simulink model "SPWM"  (R2019b)
settings: Solver=VariableStepAuto  StartTime=0.0  StopTime=1  RelTol=1e-3
InitFcn:
  | Vd = 600
libraries: powerlib_meascontrol x4
settings Model: Creator=kanth  LastModifiedBy=kanth

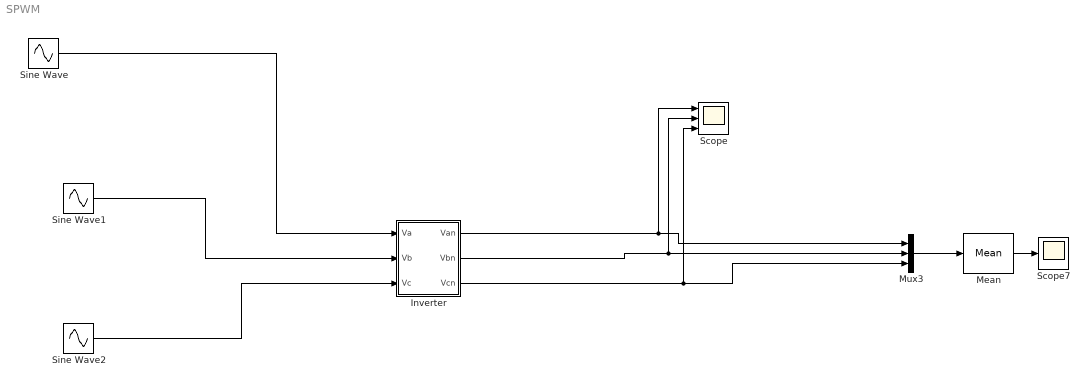
== system SPWM ==
  Inverter : Subsystem
  Mean : powerlib_meascontrol/Measurements/Mean  Freq=5000  Vinit=0  Ts=0
      settings: SourceProductName=Simscape Electrical
  Mux3 : Mux  Inputs=3
  Scope : Scope  NumInputPorts=3
  Scope7 : Scope
  Sine Wave : Sin  Amplitude=0.8  Frequency=314.159265  SampleTime=0
  Sine Wave1 : Sin  Amplitude=0.8  Frequency=314.159265  Phase=-2*pi/3  SampleTime=0
  Sine Wave2 : Sin  Amplitude=0.8  Frequency=314.159265  Phase=2*pi/3  SampleTime=0
  wires:
  Mux3/1 -> Mean/1
  Mean/1 -> Scope7/1
  Sine Wave/1 -> Inverter/1(Va)
  Sine Wave1/1 -> Inverter/2(Vb)
  Sine Wave2/1 -> Inverter/3(Vc)
  Inverter/1(Van) -> Scope/1, Mux3/1
  Inverter/2(Vbn) -> Scope/2, Mux3/2
  Inverter/3(Vcn) -> Scope/3, Mux3/3

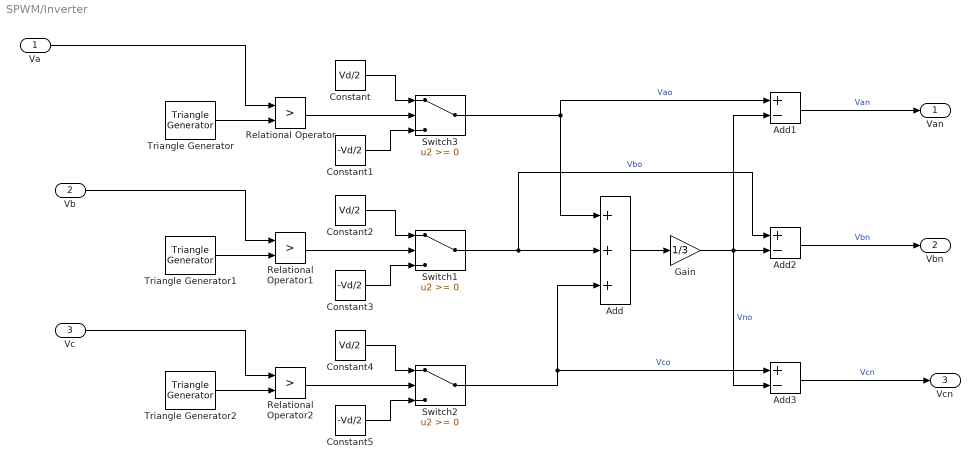
== system SPWM/Inverter ==
  Va : Inport
  Vb : Inport  Port=2
  Vc : Inport  Port=3
  Add : Sum  Inputs=+++
  Add1 : Sum  Inputs=+-
  Add2 : Sum  Inputs=+-
  Add3 : Sum  Inputs=+-
  Constant : Constant  Value=Vd/2
  Constant1 : Constant  Value=-Vd/2
  Constant2 : Constant  Value=Vd/2
  Constant3 : Constant  Value=-Vd/2
  Constant4 : Constant  Value=Vd/2
  Constant5 : Constant  Value=-Vd/2
  Gain : Gain  Gain=1/3
  Relational Operator : RelationalOperator  Operator=>  OutDataTypeStr=boolean  RndMeth=Simplest
  Relational Operator1 : RelationalOperator  Operator=>  OutDataTypeStr=boolean  RndMeth=Simplest
  Relational Operator2 : RelationalOperator  Operator=>  OutDataTypeStr=boolean  RndMeth=Simplest
  Switch1 : Switch
  Switch2 : Switch
  Switch3 : Switch
  Triangle Generator : powerlib_meascontrol/Pulse & Signal Generators/Triangle Generator  Freq=5000  Phase=0  Ts=0
      settings: SourceProductName=Simscape Electrical
  Triangle Generator1 : powerlib_meascontrol/Pulse & Signal Generators/Triangle Generator  Freq=5000  Phase=0  Ts=0
      settings: SourceProductName=Simscape Electrical
  Triangle Generator2 : powerlib_meascontrol/Pulse & Signal Generators/Triangle Generator  Freq=5000  Phase=0  Ts=0
      settings: SourceProductName=Simscape Electrical
  Van : Outport
  Vbn : Outport  Port=2
  Vcn : Outport  Port=3
  wires:
  Relational Operator1/1 -> Switch1/2
  Switch3/1 -> Add1/1, Add/1  "Vao"
  Switch1/1 -> Add/2, Add2/1  "Vbo"
  Constant2/1 -> Switch1/1
  Constant/1 -> Switch3/1
  Gain/1 -> Add3/2, Add2/2, Add1/2  "Vno"
  Constant3/1 -> Switch1/3
  Switch2/1 -> Add/3, Add3/1  "Vco"
  Relational Operator/1 -> Switch3/2
  Add3/1 -> Vcn/1  "Vcn"
  Triangle Generator/1 -> Relational Operator/2
  Triangle Generator2/1 -> Relational Operator2/2
  Constant1/1 -> Switch3/3
  Constant5/1 -> Switch2/3
  Constant4/1 -> Switch2/1
  Va/1 -> Relational Operator/1
  Add/1 -> Gain/1
  Triangle Generator1/1 -> Relational Operator1/2
  Relational Operator2/1 -> Switch2/2
  Vc/1 -> Relational Operator2/1
  Add1/1 -> Van/1  "Van"
  Vb/1 -> Relational Operator1/1
  Add2/1 -> Vbn/1  "Vbn"
